simulink model "bla"  (Simulink 6.2)
settings: Solver=ode45  StartTime=0  StopTime=0.2
libraries: simulink x2
settings Model: Creator=Admin  LastModifiedBy=sergo
settings OptimizationCC: BooleanDataType=off
settings HardwareCC: TargetUnknown=on

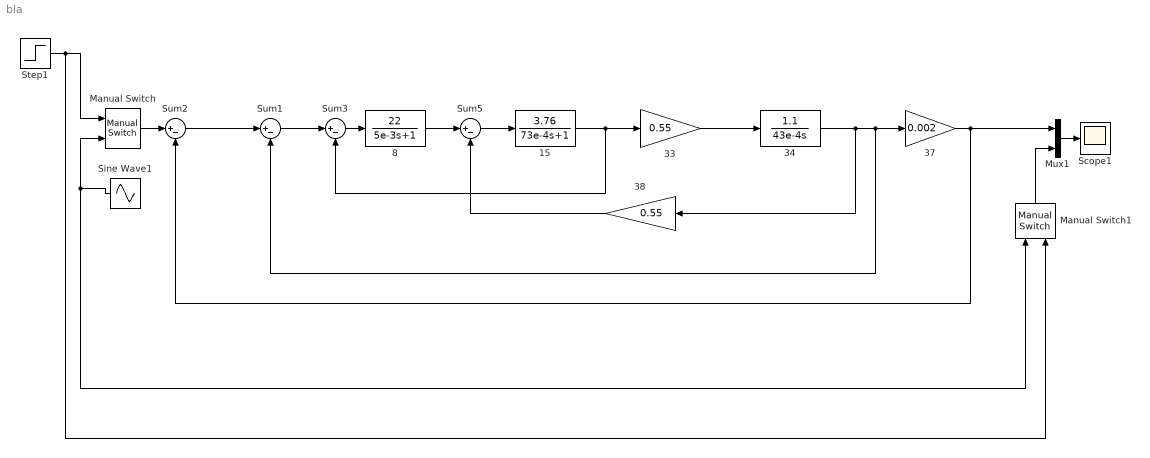
== system bla ==
  15 : TransferFcn  Numerator=[3.76]  Denominator=[73e-4 1]
  33 : Gain  Gain=0.55
  34 : TransferFcn  Numerator=[1.1]  Denominator=[43e-4 0]
  37 : Gain  Gain=0.002
  38 : Gain  Orientation=left  Gain=0.55
  8 : TransferFcn  Numerator=[22]  Denominator=[5e-3 1]
  Manual Switch : simulink/Signal Routing/Manual Switch  sw=0  action=0
  Manual Switch1 : simulink/Signal Routing/Manual Switch  Orientation=up  sw=1  action=0
  Mux1 : Mux  Inputs=2
  Scope1 : Scope
      settings: TickLabels=on  TimeRange=0.1
  Sine Wave1 : Sin  Orientation=left  Frequency=200  SampleTime=0
  Step1 : Step  Time=0  SampleTime=0
  Sum{1..3,5} (4 alike) : Sum  Inputs=|+-
  wires:
  Step1/1 -> Manual Switch/1, Manual Switch1/2
  Sine Wave1/1 -> Manual Switch/2, Manual Switch1/1
  8/1 -> Sum5/1
  Sum5/1 -> 15/1
  15/1 -> 33/1, Sum3/2
  33/1 -> 34/1
  34/1 -> 38/1, 37/1, Sum1/2
  38/1 -> Sum5/2
  Mux1/1 -> Scope1/1
  37/1 -> Mux1/1, Sum2/2
  Manual Switch1/1 -> Mux1/2
  Manual Switch/1 -> Sum2/1
  Sum3/1 -> 8/1
  Sum2/1 -> Sum1/1
  Sum1/1 -> Sum3/1
